simulink model "fig1"  (R2019b)
settings: Solver=VariableStepAuto  StartTime=0.0  StopTime=10.0  RelTol=1e-3
undefined symbols (not defined in the file): D, F, G_1, G_2, H_1, H_2, s
settings Model: Creator=jasper  LastModifiedBy=jasper

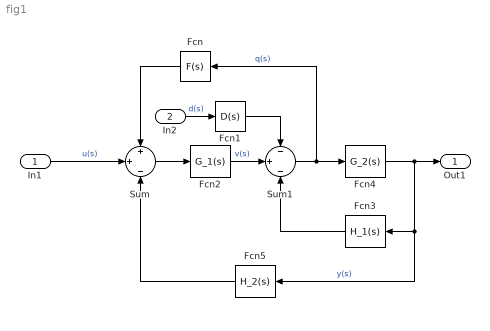
== system fig1 ==
  In1 : Inport
  In2 : Inport  Port=2
  Fcn : Fcn  Expr=F(s)
  Fcn1 : Fcn  Expr=D(s)
  Fcn2 : Fcn  Expr=G_1(s)
  Fcn3 : Fcn  Expr=H_1(s)
  Fcn4 : Fcn  Expr=G_2(s)
  Fcn5 : Fcn  Expr=H_2(s)
  Sum : Sum  Inputs=+|+|-
  Sum1 : Sum  Inputs=-|+|-
  Out1 : Outport
  wires:
  In1/1 -> Sum/2  "u(s)"
  Fcn/1 -> Sum/1
  In2/1 -> Fcn1/1  "d(s)"
  Sum/1 -> Fcn2/1
  Fcn2/1 -> Sum1/2  "v(s)"
  Fcn1/1 -> Sum1/1
  Sum1/1 -> Fcn4/1, Fcn/1  "q(s)"
  Fcn4/1 -> Fcn5/1, Fcn3/1, Out1/1  "y(s)"
  Fcn3/1 -> Sum1/3
  Fcn5/1 -> Sum/3
